simulink model "controllerDesign"  (R2023a)
settings: Solver=VariableStepAuto  StartTime=0.0  StopTime=10.0  RelTol=1e-3
undefined symbols (not defined in the file): gain, wn, zeta
settings Model: Creator=rout3  LastModifiedBy=rout3

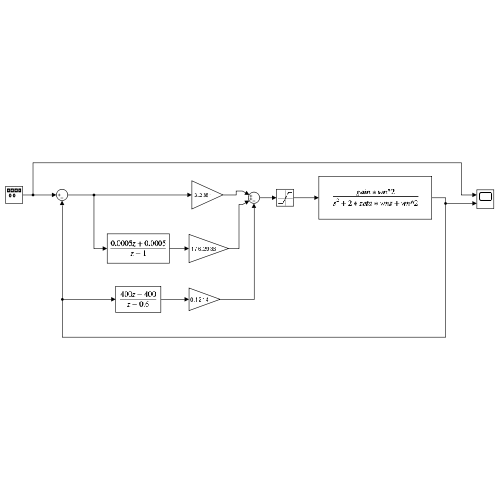
[thumbnail: Simulink's stored preview of the top-level diagram]
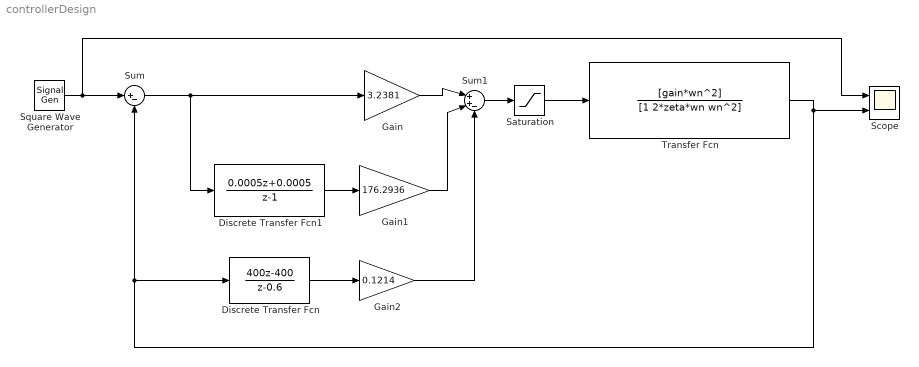
== system controllerDesign ==
  Discrete Transfer Fcn : DiscreteTransferFcn  Numerator=[400 -400]  Denominator=[1 -0.6]  SampleTime=0.001
  Discrete Transfer Fcn1 : DiscreteTransferFcn  Numerator=[0.0005 0.0005]  Denominator=[1 -1]  SampleTime=0.001
  Gain : Gain  Gain=3.2381
  Gain1 : Gain  Gain=176.2936
  Gain2 : Gain  Gain=0.1214
  Saturation : Saturate  UpperLimit=10  LowerLimit=-10
  Scope : Scope  NumInputPorts=2
  Square Wave Generator : SignalGenerator  WaveForm=square  Frequency=0.5
  Sum : Sum  Inputs=|+-
  Sum1 : Sum  Inputs=|++-
  Transfer Fcn : TransferFcn  Numerator=[gain*wn^2]  Denominator=[1 2*zeta*wn wn^2]
  wires:
  Square Wave Generator/1 -> Scope/1, Sum/1
  Sum/1 -> Discrete Transfer Fcn1/1, Gain/1
  Discrete Transfer Fcn1/1 -> Gain1/1
  Discrete Transfer Fcn/1 -> Gain2/1
  Gain2/1 -> Sum1/3
  Gain/1 -> Sum1/1
  Gain1/1 -> Sum1/2
  Sum1/1 -> Saturation/1
  Saturation/1 -> Transfer Fcn/1
  Transfer Fcn/1 -> Scope/2, Discrete Transfer Fcn/1, Sum/2
